simulink model "VCU_TDN"  (R2020a)
settings: Solver=FixedStepDiscrete  StartTime=0.0  StopTime=10.0  FixedStep=0.001  RelTol=1e-3  EnableMultiTasking=on
InitFcn:
  | EcoCoder_PreCheckLic();
undefined symbols (not defined in the file or in its folder): h, km
libraries: CoderSF_BSW_Libs x139, simulink x1, SF_CanService_Libs x1
(part 2 of 2)

== system VCU_TDN/Code/Receiving data/Inverter/Data saving/I_act_filt ==
  Data : Inport
  Enable : EnablePort
  Data Type Conversion : DataTypeConversion
  Write Measurement : CoderSF_BSW_Libs/Calibration & Measurement/Write Measurement  variable_name=I_act_filt  variable_value=0  variable_type=int16  numD=1  unitStr=""  descStr=""
      settings: AttributesFormatString=type:%<variable_type> Dimensions:%<numD>
  wires:
  Data Type Conversion/1 -> Write Measurement/1
  Data/1 -> Data Type Conversion/1

== system VCU_TDN/Code/Receiving data/Inverter/Data saving/I_cmd ==
  Data : Inport
  Enable : EnablePort
  Data Type Conversion : DataTypeConversion
  Write Measurement : CoderSF_BSW_Libs/Calibration & Measurement/Write Measurement  variable_name=I_cmd  variable_value=0  variable_type=int16  numD=1  unitStr=""  descStr=""
      settings: AttributesFormatString=type:%<variable_type> Dimensions:%<numD>
  wires:
  Data Type Conversion/1 -> Write Measurement/1
  Data/1 -> Data Type Conversion/1

== system VCU_TDN/Code/Receiving data/Inverter/Data saving/I_device ==
  Data : Inport
  Enable : EnablePort
  Data Type Conversion : DataTypeConversion
  Write Measurement : CoderSF_BSW_Libs/Calibration & Measurement/Write Measurement  variable_name=I_device  variable_value=0  variable_type=int16  numD=1  unitStr=""  descStr=""
      settings: AttributesFormatString=type:%<variable_type> Dimensions:%<numD>
  wires:
  Data Type Conversion/1 -> Write Measurement/1
  Data/1 -> Data Type Conversion/1

== system VCU_TDN/Code/Receiving data/Inverter/Data saving/I_max_eff ==
  Data : Inport
  Enable : EnablePort
  Data Type Conversion : DataTypeConversion
  Write Measurement : CoderSF_BSW_Libs/Calibration & Measurement/Write Measurement  variable_name=I_max_eff  variable_value=0  variable_type=int16  numD=1  unitStr=""  descStr=""
      settings: AttributesFormatString=type:%<variable_type> Dimensions:%<numD>
  wires:
  Data Type Conversion/1 -> Write Measurement/1
  Data/1 -> Data Type Conversion/1

== system VCU_TDN/Code/Receiving data/Inverter/Data saving/I_max_pk ==
  Data : Inport
  Enable : EnablePort
  Data Type Conversion : DataTypeConversion
  Write Measurement : CoderSF_BSW_Libs/Calibration & Measurement/Write Measurement  variable_name=I_max_pk  variable_value=0  variable_type=int16  numD=1  unitStr=""  descStr=""
      settings: AttributesFormatString=type:%<variable_type> Dimensions:%<numD>
  wires:
  Data Type Conversion/1 -> Write Measurement/1
  Data/1 -> Data Type Conversion/1

== system VCU_TDN/Code/Receiving data/Inverter/Data saving/I_nom_eff ==
  Data : Inport
  Enable : EnablePort
  Data Type Conversion : DataTypeConversion
  Write Measurement : CoderSF_BSW_Libs/Calibration & Measurement/Write Measurement  variable_name=I_nom_eff  variable_value=0  variable_type=int16  numD=1  unitStr=""  descStr=""
      settings: AttributesFormatString=type:%<variable_type> Dimensions:%<numD>
  wires:
  Data Type Conversion/1 -> Write Measurement/1
  Data/1 -> Data Type Conversion/1

== system VCU_TDN/Code/Receiving data/Inverter/Data saving/N_100 ==
  Data : Inport
  Enable : EnablePort
  Data Type Conversion : DataTypeConversion
  Write Measurement : CoderSF_BSW_Libs/Calibration & Measurement/Write Measurement  variable_name=N_100  variable_value=0  variable_type=uint16  numD=1  unitStr=""  descStr=""
      settings: AttributesFormatString=type:%<variable_type> Dimensions:%<numD>
  wires:
  Data Type Conversion/1 -> Write Measurement/1
  Data/1 -> Data Type Conversion/1

== system VCU_TDN/Code/Receiving data/Inverter/Data saving/N_Lim ==
  Data : Inport
  Enable : EnablePort
  Data Type Conversion : DataTypeConversion
  Write Measurement : CoderSF_BSW_Libs/Calibration & Measurement/Write Measurement  variable_name=N_lim  variable_value=0  variable_type=int16  numD=1  unitStr=""  descStr=""
      settings: AttributesFormatString=type:%<variable_type> Dimensions:%<numD>
  wires:
  Data Type Conversion/1 -> Write Measurement/1
  Data/1 -> Data Type Conversion/1

== system VCU_TDN/Code/Receiving data/Inverter/Data saving/N_Lim_neg ==
  Data : Inport
  Enable : EnablePort
  Data Type Conversion : DataTypeConversion
  Write Measurement : CoderSF_BSW_Libs/Calibration & Measurement/Write Measurement  variable_name=N_lim_neg  variable_value=0  variable_type=int16  numD=1  unitStr=""  descStr=""
      settings: AttributesFormatString=type:%<variable_type> Dimensions:%<numD>
  wires:
  Data Type Conversion/1 -> Write Measurement/1
  Data/1 -> Data Type Conversion/1

== system VCU_TDN/Code/Receiving data/Inverter/Data saving/N_Lim_pos ==
  Data : Inport
  Enable : EnablePort
  Data Type Conversion : DataTypeConversion
  Write Measurement : CoderSF_BSW_Libs/Calibration & Measurement/Write Measurement  variable_name=N_lim_pos  variable_value=0  variable_type=int16  numD=1  unitStr=""  descStr=""
      settings: AttributesFormatString=type:%<variable_type> Dimensions:%<numD>
  wires:
  Data Type Conversion/1 -> Write Measurement/1
  Data/1 -> Data Type Conversion/1

== system VCU_TDN/Code/Receiving data/Inverter/Data saving/N_R_Acc | M R_Acc ==
  Data : Inport
  Enable : EnablePort
  Data Type Conversion : DataTypeConversion
  Ground : Ground
  Ground1 : Ground
  Terminator : Terminator
  Write Measurement : CoderSF_BSW_Libs/Calibration & Measurement/Write Measurement  variable_name=N_R_Acc  variable_value=0  variable_type=int16  numD=1  unitStr=""  descStr=""
      settings: AttributesFormatString=type:%<variable_type> Dimensions:%<numD>
  Write Measurement1 : CoderSF_BSW_Libs/Calibration & Measurement/Write Measurement  variable_name=M_R_Acc  variable_value=0  variable_type=int16  numD=1  unitStr=""  descStr=""
      settings: AttributesFormatString=type:%<variable_type> Dimensions:%<numD>
  wires:
  Data/1 -> Data Type Conversion/1
  Data Type Conversion/1 -> Terminator/1
  Ground/1 -> Write Measurement/1
  Ground1/1 -> Write Measurement1/1

== system VCU_TDN/Code/Receiving data/Inverter/Data saving/N_R_Dec | M_R_Dec ==
  Data : Inport
  Enable : EnablePort
  Data Type Conversion : DataTypeConversion
  Ground : Ground
  Ground1 : Ground
  Terminator : Terminator
  Write Measurement : CoderSF_BSW_Libs/Calibration & Measurement/Write Measurement  variable_name=N_R_Dec  variable_value=0  variable_type=int16  numD=1  unitStr=""  descStr=""
      settings: AttributesFormatString=type:%<variable_type> Dimensions:%<numD>
  Write Measurement1 : CoderSF_BSW_Libs/Calibration & Measurement/Write Measurement  variable_name=M_R_Dec  variable_value=0  variable_type=int16  numD=1  unitStr=""  descStr=""
      settings: AttributesFormatString=type:%<variable_type> Dimensions:%<numD>
  wires:
  Data/1 -> Data Type Conversion/1
  Data Type Conversion/1 -> Terminator/1
  Ground/1 -> Write Measurement/1
  Ground1/1 -> Write Measurement1/1

== system VCU_TDN/Code/Receiving data/Inverter/Data saving/N_act_filt1 ==
  Data : Inport
  Enable : EnablePort
  Data Type Conversion : DataTypeConversion
  Write Measurement : CoderSF_BSW_Libs/Calibration & Measurement/Write Measurement  variable_name=N_act_filt  variable_value=0  variable_type=int16  numD=1  unitStr=""  descStr=""
      settings: AttributesFormatString=type:%<variable_type> Dimensions:%<numD>
  wires:
  Data Type Conversion/1 -> Write Measurement/1
  Data/1 -> Data Type Conversion/1

== system VCU_TDN/Code/Receiving data/Inverter/Data saving/SpeedRPMmax ==
  Data : Inport
  Enable : EnablePort
  Data Type Conversion : DataTypeConversion
  Write Measurement : CoderSF_BSW_Libs/Calibration & Measurement/Write Measurement  variable_name=SpeedRPMmax  variable_value=0  variable_type=int16  numD=1  unitStr=""  descStr=""
      settings: AttributesFormatString=type:%<variable_type> Dimensions:%<numD>
  wires:
  Data Type Conversion/1 -> Write Measurement/1
  Data/1 -> Data Type Conversion/1

== system VCU_TDN/Code/Receiving data/Inverter/Data saving/T_IGBT ==
  Data : Inport
  Enable : EnablePort
  Data Type Conversion : DataTypeConversion
  Write Measurement : CoderSF_BSW_Libs/Calibration & Measurement/Write Measurement  variable_name=T_IGBT  variable_value=0  variable_type=int16  numD=1  unitStr=""  descStr=""
      settings: AttributesFormatString=type:%<variable_type> Dimensions:%<numD>
  wires:
  Data Type Conversion/1 -> Write Measurement/1
  Data/1 -> Data Type Conversion/1

== system VCU_TDN/Code/Receiving data/Inverter/Data saving/T_air ==
  Data : Inport
  Enable : EnablePort
  Data Type Conversion : DataTypeConversion
  Write Measurement : CoderSF_BSW_Libs/Calibration & Measurement/Write Measurement  variable_name=T_air  variable_value=0  variable_type=int16  numD=1  unitStr=""  descStr=""
      settings: AttributesFormatString=type:%<variable_type> Dimensions:%<numD>
  wires:
  Data Type Conversion/1 -> Write Measurement/1
  Data/1 -> Data Type Conversion/1

== system VCU_TDN/Code/Receiving data/Inverter/Data saving/T_motor ==
  Data : Inport
  Enable : EnablePort
  Data Type Conversion : DataTypeConversion
  Write Measurement : CoderSF_BSW_Libs/Calibration & Measurement/Write Measurement  variable_name=T_motor  variable_value=0  variable_type=int16  numD=1  unitStr=""  descStr=""
      settings: AttributesFormatString=type:%<variable_type> Dimensions:%<numD>
  wires:
  Data Type Conversion/1 -> Write Measurement/1
  Data/1 -> Data Type Conversion/1

== system VCU_TDN/Code/Receiving data/Inverter/Data saving/Vdc_bus ==
  Data : Inport
  Enable : EnablePort
  Data Type Conversion : DataTypeConversion
  Write Measurement : CoderSF_BSW_Libs/Calibration & Measurement/Write Measurement  variable_name=Vdc_bus  variable_value=0  variable_type=int16  numD=1  unitStr=""  descStr=""
      settings: AttributesFormatString=type:%<variable_type> Dimensions:%<numD>
  wires:
  Data Type Conversion/1 -> Write Measurement/1
  Data/1 -> Data Type Conversion/1
